simulink model "Demo_TollSystem_cs"  (Simulink 7.6)
settings: Solver=FixedStepDiscrete  SolverMode=SingleTasking  StartTime=0.0  StopTime=13  FixedStep=1/20  RelTol=1e-3
model workspace (MAT data in the model file):
  mbox_table : struct (value not decoded)
  model_closed = 0
  sim_status = 0
PreLoadFcn:
  | check_NUTS_defined
  | model_closed = 0;
  | assignin('base',['model_closed_' bdroot],false);
InitFcn:
  | PreScanExperimentInitFcn(bdroot)
StopFcn:
  | PreScanExperimentStopFcn(bdroot)
libraries: simulink x9, PreScanUsefulBlocks x6, PreScanSimulinkLibrary x4
(part 1 of 2)
CloseFcn:
  | evalin('base',['clear model_closed_' bdroot]);
  | model_closed = 1;
settings Model: Creator=PRESCAN  LastModifiedBy=buildbot
settings OptimizationCC: InitFltsAndDblsToZero=on
settings DebuggingCC: SaveWithParameterizedLinksMsg=none  SignalResolutionControl=TryResolveAllWithWarning  MultiTaskDSMMsg=warning  MultiTaskCondExecSysMsg=none
settings RTWCC: IncludeERTFirstTime=on
settings GRTTargetCC: TargetFcnLib=ansi_tfl_tmw.mat

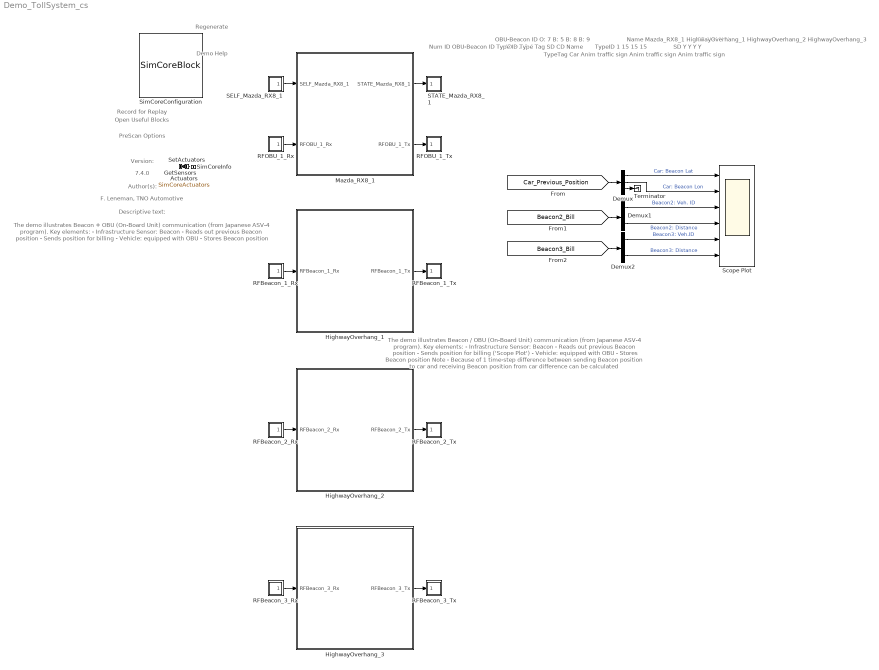
== system Demo_TollSystem_cs ==
  note: The demo illustrates Beacon / OBU (On-Board Unit)
      | communication (from Japanese ASV-4 program).
      |
      | Key elements:
      | - Infrastructure Sensor: Beacon
      |     - Reads out previous Beacon position
      |     - Sends position for billing ('Scope Plot')
      | - Vehicle: equipped with OBU
      |     - Stores Beacon position
      |
      | Note
      | - Because of 1 time-step difference between sending Beacon position
      |   to car and receiving Beacon position from car difference can be
      |   calculated
  note: Demo Help
  note: Regenerate
  note: Record for Replay
  note: Open Useful Blocks
  note: PreScan Options
  note: Version:
  note: 7.4.0
  note: Author(s):
  note: F. Leneman, TNO Automotive
  note: Descriptive text:
  note: The demo illustrates Beacon + OBU
      |
      | (On-Board Unit) communication
      | (from Japanese ASV-4 program).
      |
      | Key elements:
      | - Infrastructure Sensor: Beacon
      |     - Reads out previous Beacon
      | position
      |     - Sends position for billing
      | - Vehicle: equipped with OBU
      |     - Stores Beacon position
  note: ID
      |
      | 6
      | 2
      | 3
      | 4
  note: OBU-Beacon ID
      |
      | O: 7
      | B: 5
      | B: 8
      | B: 9
  note: TypeID
      |
      | 1
      | 15
      | 15
      | 15
  note: TypeTag
      |
      | Car
      | Anim traffic sign
      | Anim traffic sign
      | Anim traffic sign
  note: SD
      |
      | Y
      | Y
      | Y
      | Y
  note: CD
      |
      | N
      | N
      | N
      | N
  note: Name
      |
      | Mazda_RX8_1
      | HighwayOverhang_1
      | HighwayOverhang_2
      | HighwayOverhang_3
  note: Num ID OBU-Beacon ID Type ID Type Tag SD CD Name
  Actuators : DataStoreMemory  Tag=Actuators  DataStoreName=SimCoreActuators  InitialValue=zeros(79,1)
      settings: DeleteFcn=PreScanBlockDeleteFcn;
  Demux : Demux  Outputs=3
  Demux1 : Demux  Outputs=2
  Demux2 : Demux  Outputs=2
  GetSensors : Subsystem  Tag=GetSensors  Priority=2  mask(PreScan Simulation Core Block){NrOfSensors=333, TimeStep=1/20}
      mask prompts: NrOfSensors "Number of sensor values"; TimeStep "Timestep [s]"
      mask help:
      | Please do not remove this block from the PreScan compilation sheet,
      | as it contains essential configuration parameters for a PreScan simulation.
      settings: DeleteFcn=PreScanBlockDeleteFcn;
  HighwayOverhang_1 : Subsystem  Tag=WorldObjectSubSystem  InitFcn=UniqueId = '39';
      mask Display: image(imread('HighwayOverhang.jpg'));color('white');text(0,0,' ID=2\n')
  HighwayOverhang_2 : Subsystem  Tag=WorldObjectSubSystem  InitFcn=UniqueId = '40';
      mask Display: image(imread('HighwayOverhang.jpg'));color('white');text(0,0,' ID=3\n')
  HighwayOverhang_3 : Subsystem  Tag=WorldObjectSubSystem  InitFcn=|
      | UniqueId = '44';
      | UniqueId = '41';
      mask Display: image(imread('HighwayOverhang.jpg'));color('white');text(0,0,' ID=4\n')
  Mazda_RX8_1 : Subsystem  Tag=WorldObjectSubSystem  InitFcn=UniqueId = '16';
      mask Display: image(imread('Mazda_RX8.jpg'));color('white');text(0,0,' ID=6\n')
  RFBeacon_1_Rx : Subsystem  Tag=BeaconRx  Priority=3  mask(PreScan Source Block: Antenna Receiver){NrEntitiesOut=5, PortName=RFBeacon_1, PortIndex=48, PortWidth=95, TimeStep=1/20}
      mask prompts: NrEntitiesOut "User Specified: # of Visible OBUs"; PortName "Auto Assigned: Port Name [-]"; PortIndex "Auto Assigned: Index [-]"; PortWidth "Auto Assigned: Port Dimensions [-]"; TimeStep "Auto Assigned: Upload Period [s]"
      mask help:
      | Using the Beacon and OBU (On-Board Unit) information between actors and infrastructure can be exchanged.
      |
      | The Beacon Reciever receives actor information and user-definable signals.
      |
      | For more information, please click Help.
      settings: DeleteFcn=PreScanBlockDeleteFcn;
      mask Help: eval('openHelp(486)')
      mask Display: image(imread('ico_Beacon_RF_24_gray.png'))
  RFBeacon_1_Tx : Subsystem  Tag=BeaconTx  Priority=0  mask(PreScan Sink Block: AntennaT){PortName=RFBeacon_1, PortIndex=31, PortWidth=16, TimeStep=1/20}
      mask prompts: PortName "Auto Assigned: Port Name [-]"; PortIndex "Auto Assigned: Index [-]"; PortWidth "Auto Assigned: Port Dimensions [-]"; TimeStep "Auto Assigned: Upload Period [s]"
      mask help:
      | Using the Beacon and OBU (On-Board Unit) information between actors and infrastructure can be exchanged.
      |
      | The Beacon Transmitter contains the following, user-definable signals:
      |
      | - Beacon Type		[-]
      | - Spares (1:15)		[-]
      |
      | For more information, please click Help.
      settings: DeleteFcn=PreScanBlockDeleteFcn;
      mask Help: eval('openHelp(486)')
      mask Display: image(imread('ico_Beacon_RF_24_gray.png'))
  RFBeacon_2_Rx : Subsystem  Tag=BeaconRx  Priority=3  mask(PreScan Source Block: Antenna Receiver){NrEntitiesOut=5, PortName=RFBeacon_2, PortIndex=143, PortWidth=95, TimeStep=1/20}
      mask prompts: NrEntitiesOut "User Specified: # of Visible OBUs"; PortName "Auto Assigned: Port Name [-]"; PortIndex "Auto Assigned: Index [-]"; PortWidth "Auto Assigned: Port Dimensions [-]"; TimeStep "Auto Assigned: Upload Period [s]"
      mask help:
      | Using the Beacon and OBU (On-Board Unit) information between actors and infrastructure can be exchanged.
      |
      | The Beacon Reciever receives actor information and user-definable signals.
      |
      | For more information, please click Help.
      settings: DeleteFcn=PreScanBlockDeleteFcn;
      mask Help: eval('openHelp(486)')
      mask Display: image(imread('ico_Beacon_RF_24_gray.png'))
  RFBeacon_2_Tx : Subsystem  Tag=BeaconTx  Priority=0  mask(PreScan Sink Block: AntennaT){PortName=RFBeacon_2, PortIndex=47, PortWidth=16, TimeStep=1/20}
      mask prompts: PortName "Auto Assigned: Port Name [-]"; PortIndex "Auto Assigned: Index [-]"; PortWidth "Auto Assigned: Port Dimensions [-]"; TimeStep "Auto Assigned: Upload Period [s]"
      mask help:
      | Using the Beacon and OBU (On-Board Unit) information between actors and infrastructure can be exchanged.
      |
      | The Beacon Transmitter contains the following, user-definable signals:
      |
      | - Beacon Type		[-]
      | - Spares (1:15)		[-]
      |
      | For more information, please click Help.
      settings: DeleteFcn=PreScanBlockDeleteFcn;
      mask Help: eval('openHelp(486)')
      mask Display: image(imread('ico_Beacon_RF_24_gray.png'))
  RFBeacon_3_Rx : Subsystem  Tag=BeaconRx  Priority=3  mask(PreScan Source Block: Antenna Receiver){NrEntitiesOut=5, PortName=RFBeacon_3, PortIndex=238, PortWidth=95, TimeStep=1/20}
      mask prompts: NrEntitiesOut "User Specified: # of Visible OBUs"; PortName "Auto Assigned: Port Name [-]"; PortIndex "Auto Assigned: Index [-]"; PortWidth "Auto Assigned: Port Dimensions [-]"; TimeStep "Auto Assigned: Upload Period [s]"
      mask help:
      | Using the Beacon and OBU (On-Board Unit) information between actors and infrastructure can be exchanged.
      |
      | The Beacon Reciever receives actor information and user-definable signals.
      |
      | For more information, please click Help.
      settings: DeleteFcn=PreScanBlockDeleteFcn;
      mask Help: eval('openHelp(486)')
      mask Display: image(imread('ico_Beacon_RF_24_gray.png'))
  RFBeacon_3_Tx : Subsystem  Tag=BeaconTx  Priority=0  mask(PreScan Sink Block: AntennaT){PortName=RFBeacon_3, PortIndex=63, PortWidth=16, TimeStep=1/20}
      mask prompts: PortName "Auto Assigned: Port Name [-]"; PortIndex "Auto Assigned: Index [-]"; PortWidth "Auto Assigned: Port Dimensions [-]"; TimeStep "Auto Assigned: Upload Period [s]"
      mask help:
      | Using the Beacon and OBU (On-Board Unit) information between actors and infrastructure can be exchanged.
      |
      | The Beacon Transmitter contains the following, user-definable signals:
      |
      | - Beacon Type		[-]
      | - Spares (1:15)		[-]
      |
      | For more information, please click Help.
      settings: DeleteFcn=PreScanBlockDeleteFcn;
      mask Help: eval('openHelp(486)')
      mask Display: image(imread('ico_Beacon_RF_24_gray.png'))
  RFOBU_1_Rx : Subsystem  Tag=OBURx  Priority=3  mask(PreScan Source Block: Antenna Receiver){NrEntitiesOut=2, PortName=RFOBU_1, PortIndex=8, PortWidth=40, TimeStep=1/20}
      mask prompts: NrEntitiesOut "User Specified: # of Visible OBUs"; PortName "Auto Assigned: Port Name [-]"; PortIndex "Auto Assigned: Index [-]"; PortWidth "Auto Assigned: Port Dimensions [-]"; TimeStep "Auto Assigned: Upload Period [s]"
      mask help:
      | Using the Beacon and OBU (On-Board Unit) information between actors and infrastructure can be exchanged.
      |
      | The OBU Reciever receives infrastructure information and user-definable signals.
      |
      | For more information, please click Help.
      settings: DeleteFcn=PreScanBlockDeleteFcn;
      mask Help: eval('openHelp(487)')
      mask Display: image(imread('ico_OBU_RF_24_gray.png'))
  RFOBU_1_Tx : Subsystem  Tag=OBUTx  Priority=0  mask(PreScan Sink Block: AntennaT){PortName=RFOBU_1, PortIndex=15, PortWidth=16, TimeStep=1/20}
      mask prompts: PortName "Auto Assigned: Port Name [-]"; PortIndex "Auto Assigned: Index [-]"; PortWidth "Auto Assigned: Port Dimensions [-]"; TimeStep "Auto Assigned: Upload Period [s]"
      mask help:
      | Using the Beacon and OBU (On-Board Unit) information between actors and infrastructure can be exchanged.
      |
      | The OBU Transmitter contains the following, user-definable signals:
      |
      | - Vehicle Type		[-]
      | - Spares (1:15)		[-]
      |
      | For more information, please click Help.
      settings: DeleteFcn=PreScanBlockDeleteFcn;
      mask Help: eval('openHelp(487)')
      mask Display: image(imread('ico_OBU_RF_24_gray.png'))
  SELF_Mazda_RX8_1 : Subsystem  Tag=SELF  Priority=3  mask(PreScan Source Block: SELF){PortName=SELF_Mazda_RX8_1, PortIndex=0, PortWidth=8, TimeStep=1/20}
      mask prompts: PortName "Auto-Assigned: Port Name [-]"; PortIndex "Auto-Assigned: Port Index [-]"; PortWidth "Auto-Assigned: Port Dimensions"; TimeStep "Auto-Assigned: Upload Period [s]"
      mask help:
      | The SELF port shows (state) information of the actor itself. The outputs are position in the experiment's axis system and the GPS coordinates, and the object's absolute velocity and compass heading.
      |
      | For more information, please click Help.
      settings: DeleteFcn=PreScanBlockDeleteFcn;
      mask Help: eval('openHelp(462)')
      mask Display: image(imread('GPS.png'))
  STATE_Mazda_RX8_1 : Subsystem  Tag=State  Priority=0  mask(PreScan Sink Block: State){x0=-2.1430611191891602E-16, y0=-1.75, z0=0.51, Roll0=0, Pitch0=0, Yaw0=0, TimeStep=1/20}
      mask prompts: x0 "Ini x-position VEHICLE wrt GLOBAL axis system [m]"; y0 "Ini y-position VEHICLE wrt GLOBAL axis system [m]"; z0 "Ini z-position VEHICLE wrt GLOBAL axis system [m]"; Roll0 "Ini roll-angle BODY wrt VEHICLE axis system [deg]"; Pitch0 "Ini pitch-angle BODY wrt VEHICLE axis system [deg]"; Yaw0 "Ini yaw-angle VEHICLE wrt GLOBAL axis system [deg]"; TimeStep "Time Step [s]"
      mask help:
      | The Actor State contains a vector signal of size (9x1), containing the following signals:
      |
      | -  Position                  (x,y,z)                                     [m]
      | -  Velocity                  (vx,vy,vz)                               [m/s]
      | -  Angles                    (Roll, Pitch, Yaw)                   [rad]
      |
      | The Actor state is defined in the global axis system.
      | The state is superponed on the Initial position defined in the GUI.
      |
      | For more information, please click Help.
      settings: DeleteFcn=PreScanBlockDeleteFcn;
      mask Help: eval('openHelp(222)')
      mask Display: image(imread('State.png'))
  Scope Plot : Scope  NumInputPorts=6
      settings: TimeRange=14  YMin=50~5~0~0~0~0  YMax=55~5.005~200000000000000~100~200000000000000~100
  SetActuators : Subsystem  Tag=SetActuators  Priority=1  mask(PreScan Simulation Core Block){TimeStep=1/20, NrOfActuators=79}
      mask prompts: TimeStep "Timestep [s]"; NrOfActuators "Number of actuator values"
      mask help:
      | Please do not remove this block from the PreScan compilation sheet,
      | as it contains essential configuration parameters for a PreScan simulation.
      settings: DeleteFcn=PreScanBlockDeleteFcn;
  SimCoreConfiguration : M-S-Function  Tag=SimCoreConfiguration  Description=B82875A94833F997F21DD6E9124957973A9674FE07CE9C3E2714F76BA6993981  FunctionName=SimCoreBlock  Parameters=ExperimentXML PortsXML SimulationCore HostName CheckStart EnableLog RfR EnableGPUAccel ShowComputationTime  mask(PreScan Simulation Core Configurator){SimulationCore=NUTS, HostName=0, CheckStart=0, prescanversion='7.4.0', EnableLog=off, RfR=0, EnableGPUAccel=off, ShowComputationTime=off}
      mask prompts: SimulationCore "Simulation Core"; HostName "Simulation Host"; CheckStart "Show START Dialog"; prescanversion "PreScan Version"; EnableLog "Create TA Log"; RfR "Record for Replay"; EnableGPUAccel "Enable GPU Acceleration"; ShowComputationTime "Show ComputationTime Scope"
      mask help:
      | Please do not remove this block from the PreScan compilation sheet,
      | as it contains essential configuration parameter for a PreScan simulation.
      mask init:
      | model = bdroot;
      | ExperimentXML = [model(1:end-3) '.pex'];
      | PortsXML = [model '_ports.pcd'];
      settings: DeleteFcn=PreScanBlockDeleteFcn;  ModelCloseFcn=assignin('base',['model_closed_' bdroot],true);
      mask Help: eval('openHelp(812)')
      mask Display: image(imread('prescanlogo.ico'))
  SimCoreInfo : Subsystem  Tag=SimCoreInfo
  Terminator : Terminator
  wires:
  [Car_Previous_Position] -> Demux/1
  Demux/3 -> Terminator/1
  Demux/1 -> Scope Plot/1  "Car: Beacon Lat"
  Demux/2 -> Scope Plot/2  "Car: Beacon Lon"
  [Beacon2_Bill] -> Demux1/1
  Demux1/1 -> Scope Plot/3  "Beacon2: Veh. ID"
  Demux1/2 -> Scope Plot/4  "Beacon2: Distance"
  [Beacon3_Bill] -> Demux2/1
  Demux2/1 -> Scope Plot/5  "Beacon3: Veh.ID"
  Demux2/2 -> Scope Plot/6  "Beacon3: Distance"
  Mazda_RX8_1/1(STATE_Mazda_RX8_1) -> STATE_Mazda_RX8_1/1(State)
  SELF_Mazda_RX8_1/1(U) -> Mazda_RX8_1/1(SELF_Mazda_RX8_1)
  RFOBU_1_Rx/1(U) -> Mazda_RX8_1/2(RFOBU_1_Rx)
  Mazda_RX8_1/2(RFOBU_1_Tx) -> RFOBU_1_Tx/1(Y)
  RFBeacon_1_Rx/1(U) -> HighwayOverhang_1/1(RFBeacon_1_Rx)
  HighwayOverhang_1/1(RFBeacon_1_Tx) -> RFBeacon_1_Tx/1(Y)
  RFBeacon_2_Rx/1(U) -> HighwayOverhang_2/1(RFBeacon_2_Rx)
  HighwayOverhang_2/1(RFBeacon_2_Tx) -> RFBeacon_2_Tx/1(Y)
  RFBeacon_3_Rx/1(U) -> HighwayOverhang_3/1(RFBeacon_3_Rx)
  HighwayOverhang_3/1(RFBeacon_3_Tx) -> RFBeacon_3_Tx/1(Y)
  SetActuators/1(dummy) -> GetSensors/1(dummy)

== system Demo_TollSystem_cs/GetSensors ==
  dummy : Inport
  GetSensors : M-S-Function  FunctionName=GetSensorsBlock  Parameters=TimeStep NrOfSensors
  tag scope: SimCoreSensors=global
  wires:
  GetSensors/1 -> [SimCoreSensors]
  dummy/1 -> GetSensors/1

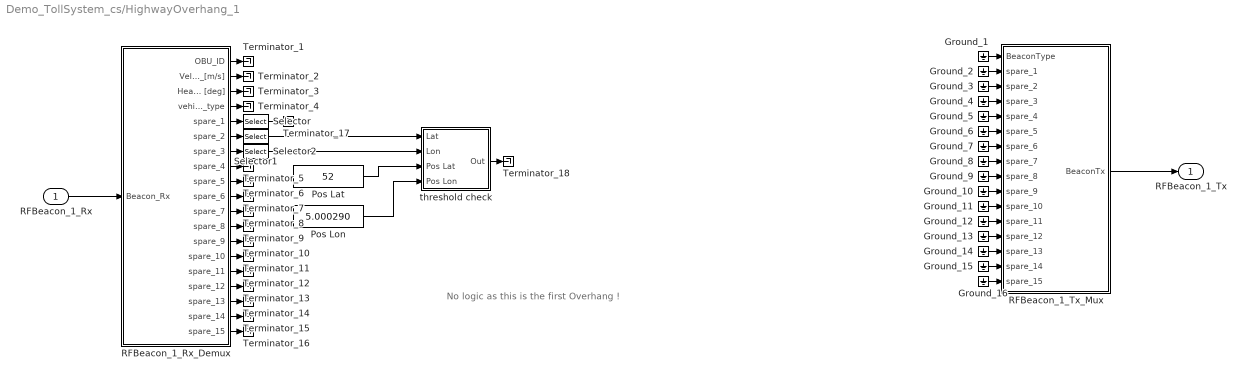
== system Demo_TollSystem_cs/HighwayOverhang_1 ==
  note: No logic as this is the first Overhang !
  RFBeacon_1_Rx : Inport  Tag=BeaconRxInport
  Ground_{1..16} (16 alike) : Ground
  Pos Lat : Constant  Value=52
  Pos Lon : Constant  Value=5.000290
  RFBeacon_1_Rx_Demux : Subsystem  Tag=DemuxAntennaR  mask(PreScan Demux Block:){Technology='RF'}
      mask init:
      | IconTxt = char('','','','','Technology:            ',['{\it',Technology,'}']);
      settings: DeleteFcn=PreScanBlockDeleteFcn;
      mask Display:
      | disp(IconTxt,'texmode','on')
      | port_label('output', 1, 'OBU ID [-]')
      | port_label('output', 2, 'OBU Velocity [m/s]')
      | port_label('output', 3, 'OBU Heading [deg]')
      | port_label('output', 4, 'Vehicle Type[-]')
      | port_label('output', 5, 'Veh. Reg.')
      | port_label('output', 6, 'Previous pos. - Lat')
      | port_label('output', 7, 'Previous pos. - Lon')
      | port_label('output', 8, 'Previous pos. - Alt')
      | port_label('output', 9, 'spare_5')
      | port_label('output', 10, 'spare_6')
      | port_label('output', 11, 'spare_7')
      | port_label('output', 12, 'spare_8')
      | port_label('output', 13, 'spare_9')
      | port_label('output', 14, 'spare_10')
      | port_label('output', 15, 'spare_11')
      | port_label('output', 16, 'spare_12')
      | port_label('output', 17, 'spare_13')
      | port_label('output', 18, 'spare_14')
      | port_label('output', 19, 'spare_15')
  RFBeacon_1_Tx_Mux : Subsystem  Tag=MuxBeaconTx  mask(PreScan Mux Block:){Technology='RF'}
      mask init:
      | IconTxt = char('','','','              Technology:',['{\it                ',Technology,'}']);
      settings: DeleteFcn=PreScanBlockDeleteFcn;
      mask Display:
      | disp(IconTxt,'texmode','on')
      | port_label('input', 1, 'Beacon Type [-]')
      | port_label('input', 2, 'spare_1')
      | port_label('input', 3, 'spare_2')
      | port_label('input', 4, 'spare_3')
      | port_label('input', 5, 'spare_4')
      | port_label('input', 6, 'spare_5')
      | port_label('input', 7, 'spare_6')
      | port_label('input', 8, 'spare_7')
      | port_label('input', 9, 'spare_8')
      | port_label('input', 10, 'spare_9')
      | port_label('input', 11, 'spare_10')
      | port_label('input', 12, 'spare_11')
      | port_label('input', 13, 'spare_12')
      | port_label('input', 14, 'spare_13')
      | port_label('input', 15, 'spare_14')
      | port_label('input', 16, 'spare_15')
  Selector : Selector  IndexOptions=Index vector (dialog)  Indices=[1]  OutputSizes=1
  Selector1 : Selector  IndexOptions=Index vector (dialog)  Indices=[1]  OutputSizes=1
  Selector2 : Selector  IndexOptions=Index vector (dialog)  Indices=[1]  OutputSizes=1
  Terminator_{1..18} (18 alike) : Terminator
  threshold check : Subsystem
  RFBeacon_1_Tx : Outport  Tag=AntennaTOutport
  wires:
  Selector1/1 -> threshold check/1(Lat)
  Selector2/1 -> threshold check/2(Lon)
  Pos Lat/1 -> threshold check/3(Pos Lat)
  Pos Lon/1 -> threshold check/4(Pos Lon)
  RFBeacon_1_Rx/1 -> RFBeacon_1_Rx_Demux/1(Beacon_Rx)
  RFBeacon_1_Tx_Mux/1(BeaconTx) -> RFBeacon_1_Tx/1
  RFBeacon_1_Rx_Demux/5(spare_1) -> Selector/1
  RFBeacon_1_Rx_Demux/6(spare_2) -> Selector1/1
  RFBeacon_1_Rx_Demux/7(spare_3) -> Selector2/1
  RFBeacon_1_Rx_Demux/1(OBU_ID) -> Terminator_1/1
  RFBeacon_1_Rx_Demux/2(Velocity_[m/s]) -> Terminator_2/1
  RFBeacon_1_Rx_Demux/3(Heading [deg]) -> Terminator_3/1
  RFBeacon_1_Rx_Demux/4(vehicle_type) -> Terminator_4/1
  RFBeacon_1_Rx_Demux/8(spare_4) -> Terminator_5/1
  RFBeacon_1_Rx_Demux/9(spare_5) -> Terminator_6/1
  RFBeacon_1_Rx_Demux/10(spare_6) -> Terminator_7/1
  RFBeacon_1_Rx_Demux/11(spare_7) -> Terminator_8/1
  RFBeacon_1_Rx_Demux/12(spare_8) -> Terminator_9/1
  RFBeacon_1_Rx_Demux/13(spare_9) -> Terminator_10/1
  RFBeacon_1_Rx_Demux/14(spare_10) -> Terminator_11/1
  RFBeacon_1_Rx_Demux/15(spare_11) -> Terminator_12/1
  RFBeacon_1_Rx_Demux/16(spare_12) -> Terminator_13/1
  RFBeacon_1_Rx_Demux/17(spare_13) -> Terminator_14/1
  RFBeacon_1_Rx_Demux/18(spare_14) -> Terminator_15/1
  RFBeacon_1_Rx_Demux/19(spare_15) -> Terminator_16/1
  Ground_1/1 -> RFBeacon_1_Tx_Mux/1(BeaconType)
  Ground_2/1 -> RFBeacon_1_Tx_Mux/2(spare_1)
  Ground_3/1 -> RFBeacon_1_Tx_Mux/3(spare_2)
  Ground_4/1 -> RFBeacon_1_Tx_Mux/4(spare_3)
  Ground_5/1 -> RFBeacon_1_Tx_Mux/5(spare_4)
  Ground_6/1 -> RFBeacon_1_Tx_Mux/6(spare_5)
  Ground_7/1 -> RFBeacon_1_Tx_Mux/7(spare_6)
  Ground_8/1 -> RFBeacon_1_Tx_Mux/8(spare_7)
  Ground_9/1 -> RFBeacon_1_Tx_Mux/9(spare_8)
  Ground_10/1 -> RFBeacon_1_Tx_Mux/10(spare_9)
  Ground_11/1 -> RFBeacon_1_Tx_Mux/11(spare_10)
  Ground_12/1 -> RFBeacon_1_Tx_Mux/12(spare_11)
  Ground_13/1 -> RFBeacon_1_Tx_Mux/13(spare_12)
  Ground_14/1 -> RFBeacon_1_Tx_Mux/14(spare_13)
  Ground_15/1 -> RFBeacon_1_Tx_Mux/15(spare_14)
  Ground_16/1 -> RFBeacon_1_Tx_Mux/16(spare_15)
  Selector/1 -> Terminator_17/1
  threshold check/1(Out) -> Terminator_18/1

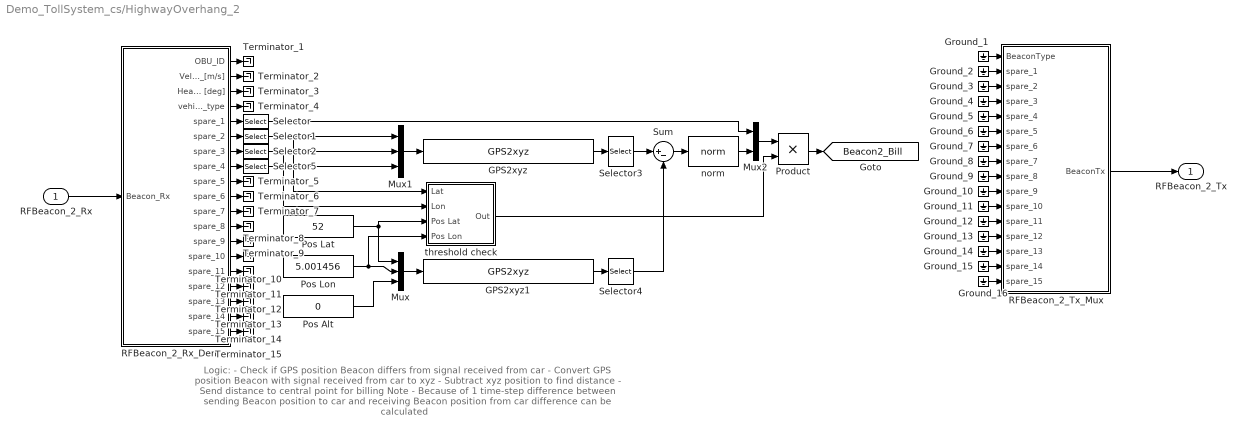
== system Demo_TollSystem_cs/HighwayOverhang_2 ==
  note: Logic:
      | - Check if GPS position Beacon differs from signal received from car
      | - Convert GPS position Beacon with signal received from car to xyz
      | - Subtract xyz position to find distance
      | - Send distance to central point for billing
      |
      | Note
      | - Because of 1 time-step difference between sending Beacon position
      |   to car and receiving Beacon position from car difference can be
      |   calculated
  RFBeacon_2_Rx : Inport  Tag=BeaconRxInport
  GPS2xyz : PreScanUsefulBlocks/GPS2xyz  CoordinateCount=1  GPS_base=[52 5 0]
  GPS2xyz1 : PreScanUsefulBlocks/GPS2xyz  CoordinateCount=1  GPS_base=[52 5 0]
  Ground_{1..16} (16 alike) : Ground
  Mux : Mux  Inputs=3
  Mux1 : Mux  Inputs=3
  Mux2 : Mux  Inputs=2
  Pos Alt : Constant  Value=0
  Pos Lat : Constant  Value=52
  Pos Lon : Constant  Value=5.001456
  Product : Product  RndMeth=Zero
  RFBeacon_2_Rx_Demux : Subsystem  Tag=DemuxAntennaR  mask(PreScan Demux Block:){Technology='RF'}
      mask init:
      | IconTxt = char('','','','','Technology:            ',['{\it',Technology,'}']);
      settings: DeleteFcn=PreScanBlockDeleteFcn;
      mask Display:
      | disp(IconTxt,'texmode','on')
      | port_label('output', 1, 'OBU ID [-]')
      | port_label('output', 2, 'OBU Velocity [m/s]')
      | port_label('output', 3, 'OBU Heading [deg]')
      | port_label('output', 4, 'Vehicle Type[-]')
      | port_label('output', 5, 'Veh. Reg.')
      | port_label('output', 6, 'Previous pos. - Lat')
      | port_label('output', 7, 'Previous pos. - Lon')
      | port_label('output', 8, 'Previous pos. - Alt')
      | port_label('output', 9, 'spare_5')
      | port_label('output', 10, 'spare_6')
      | port_label('output', 11, 'spare_7')
      | port_label('output', 12, 'spare_8')
      | port_label('output', 13, 'spare_9')
      | port_label('output', 14, 'spare_10')
      | port_label('output', 15, 'spare_11')
      | port_label('output', 16, 'spare_12')
      | port_label('output', 17, 'spare_13')
      | port_label('output', 18, 'spare_14')
      | port_label('output', 19, 'spare_15')
  RFBeacon_2_Tx_Mux : Subsystem  Tag=MuxBeaconTx  mask(PreScan Mux Block:){Technology='RF'}
      mask init:
      | IconTxt = char('','','','              Technology:',['{\it                ',Technology,'}']);
      settings: DeleteFcn=PreScanBlockDeleteFcn;
      mask Display:
      | disp(IconTxt,'texmode','on')
      | port_label('input', 1, 'Beacon Type [-]')
      | port_label('input', 2, 'spare_1')
      | port_label('input', 3, 'spare_2')
      | port_label('input', 4, 'spare_3')
      | port_label('input', 5, 'spare_4')
      | port_label('input', 6, 'spare_5')
      | port_label('input', 7, 'spare_6')
      | port_label('input', 8, 'spare_7')
      | port_label('input', 9, 'spare_8')
      | port_label('input', 10, 'spare_9')
      | port_label('input', 11, 'spare_10')
      | port_label('input', 12, 'spare_11')
      | port_label('input', 13, 'spare_12')
      | port_label('input', 14, 'spare_13')
      | port_label('input', 15, 'spare_14')
      | port_label('input', 16, 'spare_15')
  Selector{,1..2,5} (4 alike) : Selector  IndexOptions=Index vector (dialog)  Indices=[1]  OutputSizes=1
  Selector3 : Selector  InputPortWidth=3  IndexOptions=Index vector (dialog)  Indices=[1 2]  OutputSizes=1
  Selector4 : Selector  InputPortWidth=3  IndexOptions=Index vector (dialog)  Indices=[1 2]  OutputSizes=1
  Sum : Sum  Inputs=|+-
  Terminator_{1..15} (15 alike) : Terminator
  norm : MATLABFcn  MATLABFcn=norm
  threshold check : Subsystem
  RFBeacon_2_Tx : Outport  Tag=AntennaTOutport
  tag scope: Beacon2_Bill=global
  wires:
  threshold check/1(Out) -> Product/2
  Pos Lat/1 -> threshold check/3(Pos Lat), Mux/1
  Pos Lon/1 -> threshold check/4(Pos Lon), Mux/2
  Pos Alt/1 -> Mux/3
  Selector/1 -> Mux2/1
  Selector1/1 -> threshold check/1(Lat), Mux1/1
  Selector2/1 -> Mux1/2, threshold check/2(Lon)
  Mux1/1 -> GPS2xyz/1
  Mux/1 -> GPS2xyz1/1
  GPS2xyz/1 -> Selector3/1
  GPS2xyz1/1 -> Selector4/1
  Selector3/1 -> Sum/1
  Selector4/1 -> Sum/2
  Sum/1 -> norm/1
  Selector5/1 -> Mux1/3
  norm/1 -> Mux2/2
  Mux2/1 -> Product/1
  Product/1 -> [Beacon2_Bill]
  RFBeacon_2_Rx/1 -> RFBeacon_2_Rx_Demux/1(Beacon_Rx)
  RFBeacon_2_Tx_Mux/1(BeaconTx) -> RFBeacon_2_Tx/1
  RFBeacon_2_Rx_Demux/5(spare_1) -> Selector/1
  RFBeacon_2_Rx_Demux/6(spare_2) -> Selector1/1
  RFBeacon_2_Rx_Demux/7(spare_3) -> Selector2/1
  RFBeacon_2_Rx_Demux/8(spare_4) -> Selector5/1
  RFBeacon_2_Rx_Demux/1(OBU_ID) -> Terminator_1/1
  RFBeacon_2_Rx_Demux/2(Velocity_[m/s]) -> Terminator_2/1
  RFBeacon_2_Rx_Demux/3(Heading [deg]) -> Terminator_3/1
  RFBeacon_2_Rx_Demux/4(vehicle_type) -> Terminator_4/1
  RFBeacon_2_Rx_Demux/9(spare_5) -> Terminator_5/1
  RFBeacon_2_Rx_Demux/10(spare_6) -> Terminator_6/1
  RFBeacon_2_Rx_Demux/11(spare_7) -> Terminator_7/1
  RFBeacon_2_Rx_Demux/12(spare_8) -> Terminator_8/1
  RFBeacon_2_Rx_Demux/13(spare_9) -> Terminator_9/1
  RFBeacon_2_Rx_Demux/14(spare_10) -> Terminator_10/1
  RFBeacon_2_Rx_Demux/15(spare_11) -> Terminator_11/1
  RFBeacon_2_Rx_Demux/16(spare_12) -> Terminator_12/1
  RFBeacon_2_Rx_Demux/17(spare_13) -> Terminator_13/1
  RFBeacon_2_Rx_Demux/18(spare_14) -> Terminator_14/1
  RFBeacon_2_Rx_Demux/19(spare_15) -> Terminator_15/1
  Ground_1/1 -> RFBeacon_2_Tx_Mux/1(BeaconType)
  Ground_2/1 -> RFBeacon_2_Tx_Mux/2(spare_1)
  Ground_3/1 -> RFBeacon_2_Tx_Mux/3(spare_2)
  Ground_4/1 -> RFBeacon_2_Tx_Mux/4(spare_3)
  Ground_5/1 -> RFBeacon_2_Tx_Mux/5(spare_4)
  Ground_6/1 -> RFBeacon_2_Tx_Mux/6(spare_5)
  Ground_7/1 -> RFBeacon_2_Tx_Mux/7(spare_6)
  Ground_8/1 -> RFBeacon_2_Tx_Mux/8(spare_7)
  Ground_9/1 -> RFBeacon_2_Tx_Mux/9(spare_8)
  Ground_10/1 -> RFBeacon_2_Tx_Mux/10(spare_9)
  Ground_11/1 -> RFBeacon_2_Tx_Mux/11(spare_10)
  Ground_12/1 -> RFBeacon_2_Tx_Mux/12(spare_11)
  Ground_13/1 -> RFBeacon_2_Tx_Mux/13(spare_12)
  Ground_14/1 -> RFBeacon_2_Tx_Mux/14(spare_13)
  Ground_15/1 -> RFBeacon_2_Tx_Mux/15(spare_14)
  Ground_16/1 -> RFBeacon_2_Tx_Mux/16(spare_15)

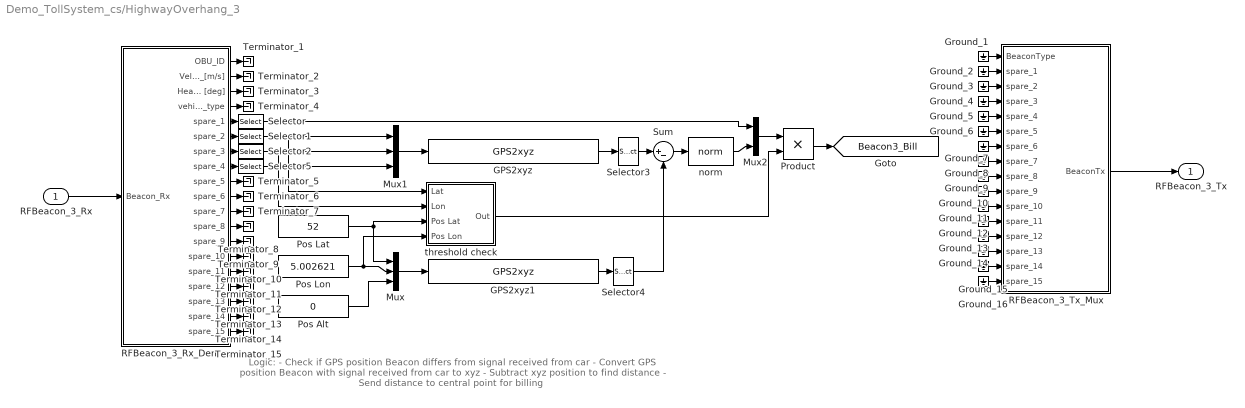
== system Demo_TollSystem_cs/HighwayOverhang_3 ==
  note: Logic:
      | - Check if GPS position Beacon differs from signal received from car
      | - Convert GPS position Beacon with signal received from car to xyz
      | - Subtract xyz position to find distance
      | - Send distance to central point for billing
  RFBeacon_3_Rx : Inport  Tag=BeaconRxInport
  GPS2xyz : PreScanUsefulBlocks/GPS2xyz  CoordinateCount=1  GPS_base=[52 5 0]
  GPS2xyz1 : PreScanUsefulBlocks/GPS2xyz  CoordinateCount=1  GPS_base=[52 5 0]
  Ground_{1..16} (16 alike) : Ground
  Mux : Mux  Inputs=3
  Mux1 : Mux  Inputs=3
  Mux2 : Mux  Inputs=2
  Pos Alt : Constant  Value=0
  Pos Lat : Constant  Value=52
  Pos Lon : Constant  Value=5.002621
  Product : Product  RndMeth=Zero
  RFBeacon_3_Rx_Demux : Subsystem  Tag=DemuxAntennaR  mask(PreScan Demux Block:){Technology='RF'}
      mask init:
      | IconTxt = char('','','','','Technology:            ',['{\it',Technology,'}']);
      settings: DeleteFcn=PreScanBlockDeleteFcn;
      mask Display:
      | disp(IconTxt,'texmode','on')
      | port_label('output', 1, 'OBU ID [-]')
      | port_label('output', 2, 'OBU Velocity [m/s]')
      | port_label('output', 3, 'OBU Heading [deg]')
      | port_label('output', 4, 'Vehicle Type[-]')
      | port_label('output', 5, 'Veh. Reg.')
      | port_label('output', 6, 'Previous pos. - Lat')
      | port_label('output', 7, 'Previous pos. - Lon')
      | port_label('output', 8, 'Previous pos. - Alt')
      | port_label('output', 9, 'spare_5')
      | port_label('output', 10, 'spare_6')
      | port_label('output', 11, 'spare_7')
      | port_label('output', 12, 'spare_8')
      | port_label('output', 13, 'spare_9')
      | port_label('output', 14, 'spare_10')
      | port_label('output', 15, 'spare_11')
      | port_label('output', 16, 'spare_12')
      | port_label('output', 17, 'spare_13')
      | port_label('output', 18, 'spare_14')
      | port_label('output', 19, 'spare_15')
  RFBeacon_3_Tx_Mux : Subsystem  Tag=MuxBeaconTx  mask(PreScan Mux Block:){Technology='RF'}
      mask init:
      | IconTxt = char('','','','              Technology:',['{\it                ',Technology,'}']);
      settings: DeleteFcn=PreScanBlockDeleteFcn;
      mask Display:
      | disp(IconTxt,'texmode','on')
      | port_label('input', 1, 'Beacon Type [-]')
      | port_label('input', 2, 'spare_1')
      | port_label('input', 3, 'spare_2')
      | port_label('input', 4, 'spare_3')
      | port_label('input', 5, 'spare_4')
      | port_label('input', 6, 'spare_5')
      | port_label('input', 7, 'spare_6')
      | port_label('input', 8, 'spare_7')
      | port_label('input', 9, 'spare_8')
      | port_label('input', 10, 'spare_9')
      | port_label('input', 11, 'spare_10')
      | port_label('input', 12, 'spare_11')
      | port_label('input', 13, 'spare_12')
      | port_label('input', 14, 'spare_13')
      | port_label('input', 15, 'spare_14')
      | port_label('input', 16, 'spare_15')
  Selector{,1..2,5} (4 alike) : Selector  IndexOptions=Index vector (dialog)  Indices=[1]  OutputSizes=1
  Selector3 : Selector  InputPortWidth=3  IndexOptions=Index vector (dialog)  Indices=[1 2]  OutputSizes=1
  Selector4 : Selector  InputPortWidth=3  IndexOptions=Index vector (dialog)  Indices=[1 2]  OutputSizes=1
  Sum : Sum  Inputs=|+-
  Terminator_{1..15} (15 alike) : Terminator
  norm : MATLABFcn  MATLABFcn=norm
  threshold check : Subsystem
  RFBeacon_3_Tx : Outport  Tag=AntennaTOutport
  tag scope: Beacon3_Bill=global
  wires:
  threshold check/1(Out) -> Product/2
  Pos Lat/1 -> threshold check/3(Pos Lat), Mux/1
  Pos Lon/1 -> threshold check/4(Pos Lon), Mux/2
  Pos Alt/1 -> Mux/3
  Selector/1 -> Mux2/1
  Selector1/1 -> threshold check/1(Lat), Mux1/1
  Selector2/1 -> Mux1/2, threshold check/2(Lon)
  Mux1/1 -> GPS2xyz/1
  Mux/1 -> GPS2xyz1/1
  GPS2xyz/1 -> Selector3/1
  GPS2xyz1/1 -> Selector4/1
  Selector3/1 -> Sum/1
  Selector4/1 -> Sum/2
  Sum/1 -> norm/1
  Selector5/1 -> Mux1/3
  norm/1 -> Mux2/2
  Mux2/1 -> Product/1
  Product/1 -> [Beacon3_Bill]
  RFBeacon_3_Rx/1 -> RFBeacon_3_Rx_Demux/1(Beacon_Rx)
  RFBeacon_3_Tx_Mux/1(BeaconTx) -> RFBeacon_3_Tx/1
  RFBeacon_3_Rx_Demux/5(spare_1) -> Selector/1
  RFBeacon_3_Rx_Demux/6(spare_2) -> Selector1/1
  RFBeacon_3_Rx_Demux/7(spare_3) -> Selector2/1
  RFBeacon_3_Rx_Demux/8(spare_4) -> Selector5/1
  RFBeacon_3_Rx_Demux/1(OBU_ID) -> Terminator_1/1
  RFBeacon_3_Rx_Demux/2(Velocity_[m/s]) -> Terminator_2/1
  RFBeacon_3_Rx_Demux/3(Heading [deg]) -> Terminator_3/1
  RFBeacon_3_Rx_Demux/4(vehicle_type) -> Terminator_4/1
  RFBeacon_3_Rx_Demux/9(spare_5) -> Terminator_5/1
  RFBeacon_3_Rx_Demux/10(spare_6) -> Terminator_6/1
  RFBeacon_3_Rx_Demux/11(spare_7) -> Terminator_7/1
  RFBeacon_3_Rx_Demux/12(spare_8) -> Terminator_8/1
  RFBeacon_3_Rx_Demux/13(spare_9) -> Terminator_9/1
  RFBeacon_3_Rx_Demux/14(spare_10) -> Terminator_10/1
  RFBeacon_3_Rx_Demux/15(spare_11) -> Terminator_11/1
  RFBeacon_3_Rx_Demux/16(spare_12) -> Terminator_12/1
  RFBeacon_3_Rx_Demux/17(spare_13) -> Terminator_13/1
  RFBeacon_3_Rx_Demux/18(spare_14) -> Terminator_14/1
  RFBeacon_3_Rx_Demux/19(spare_15) -> Terminator_15/1
  Ground_1/1 -> RFBeacon_3_Tx_Mux/1(BeaconType)
  Ground_2/1 -> RFBeacon_3_Tx_Mux/2(spare_1)
  Ground_3/1 -> RFBeacon_3_Tx_Mux/3(spare_2)
  Ground_4/1 -> RFBeacon_3_Tx_Mux/4(spare_3)
  Ground_5/1 -> RFBeacon_3_Tx_Mux/5(spare_4)
  Ground_6/1 -> RFBeacon_3_Tx_Mux/6(spare_5)
  Ground_7/1 -> RFBeacon_3_Tx_Mux/7(spare_6)
  Ground_8/1 -> RFBeacon_3_Tx_Mux/8(spare_7)
  Ground_9/1 -> RFBeacon_3_Tx_Mux/9(spare_8)
  Ground_10/1 -> RFBeacon_3_Tx_Mux/10(spare_9)
  Ground_11/1 -> RFBeacon_3_Tx_Mux/11(spare_10)
  Ground_12/1 -> RFBeacon_3_Tx_Mux/12(spare_11)
  Ground_13/1 -> RFBeacon_3_Tx_Mux/13(spare_12)
  Ground_14/1 -> RFBeacon_3_Tx_Mux/14(spare_13)
  Ground_15/1 -> RFBeacon_3_Tx_Mux/15(spare_14)
  Ground_16/1 -> RFBeacon_3_Tx_Mux/16(spare_15)

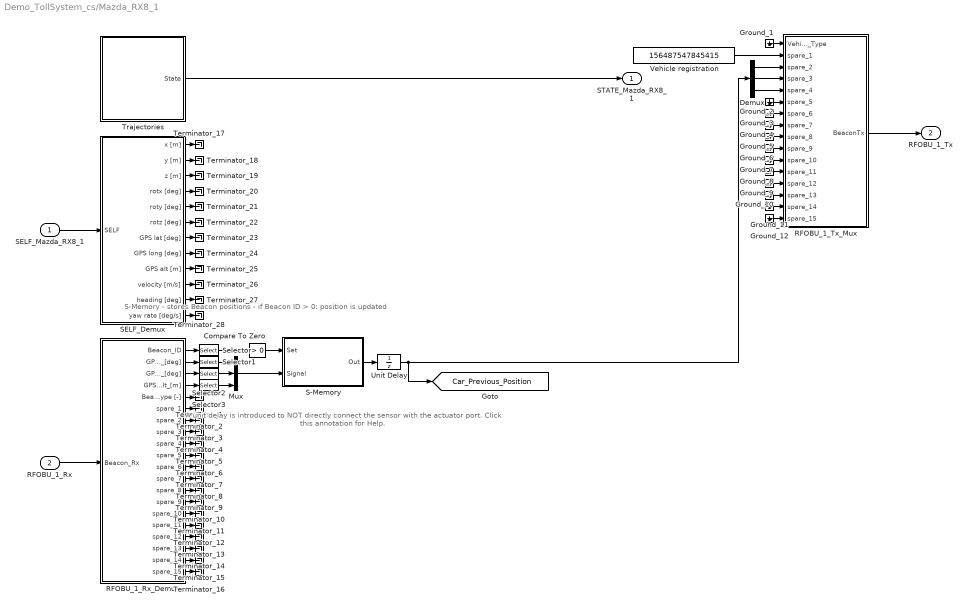
== system Demo_TollSystem_cs/Mazda_RX8_1 ==
  note: A unit delay is introduced to NOT
      | directly connect the sensor with
      | the actuator port.
      |
      | Click this annotation for Help.
  note: S-Memory
      | - stores Beacon positions
      | - if Beacon ID > 0: position is updated
  SELF_Mazda_RX8_1 : Inport  Tag=SELFInport
  RFOBU_1_Rx : Inport  Tag=OBURxInport  Port=2
  Compare To Zero : simulink/Logic and Bit Operations/Compare To Zero  SystemSampleTime=-1  relop=>  LogicOutDataTypeMode=uint8  ZeroCross=off
  Demux : Demux  Outputs=3
  Ground_{1..12} (12 alike) : Ground
  Mux : Mux  Inputs=3
  RFOBU_1_Rx_Demux : Subsystem  Tag=DemuxOBURx  mask(PreScan Demux Block:){Technology='RF'}
      mask init:
      | IconTxt = char('','','','Technology:            ',['{\it',Technology,'}']);
      settings: DeleteFcn=PreScanBlockDeleteFcn;
      mask Display:
      | disp(IconTxt,'texmode','on')
      | port_label('output', 1, 'Beacon ID [-]')
      | port_label('output', 2, 'Beacon GPS Lat [deg]')
      | port_label('output', 3, 'Beacon GPS Lon [deg]')
      | port_label('output', 4, 'Beacon GPS Alt [m]')
      | port_label('output', 5, 'BeaconType [-]')
      | port_label('output', 6, 'spare_1')
      | port_label('output', 7, 'spare_2')
      | port_label('output', 8, 'spare_3')
      | port_label('output', 9, 'spare_4')
      | port_label('output', 10, 'spare_5')
      | port_label('output', 11, 'spare_6')
      | port_label('output', 12, 'spare_7')
      | port_label('output', 13, 'spare_8')
      | port_label('output', 14, 'spare_9')
      | port_label('output', 15, 'spare_10')
      | port_label('output', 16, 'spare_11')
      | port_label('output', 17, 'spare_12')
      | port_label('output', 18, 'spare_13')
      | port_label('output', 19, 'spare_14')
      | port_label('output', 20, 'spare_15')
  RFOBU_1_Tx_Mux : Subsystem  Tag=MuxOBUTx  mask(PreScan Mux Block:){Technology='RF'}
      mask init:
      | IconTxt = char('','','              Technology:',['{\it                ',Technology,'}']);
      settings: DeleteFcn=PreScanBlockDeleteFcn;
      mask Display:
      | disp(IconTxt,'texmode','on')
      | port_label('input', 1, 'Vehicle Type [-]')
      | port_label('input', 2, 'Veh. Reg.')
      | port_label('input', 3, 'Previous pos. - Lat')
      | port_label('input', 4, 'Previous pos. - Lon')
      | port_label('input', 5, 'Previous pos. - Alt')
      | port_label('input', 6, 'spare_5')
      | port_label('input', 7, 'spare_6')
      | port_label('input', 8, 'spare_7')
      | port_label('input', 9, 'spare_8')
      | port_label('input', 10, 'spare_9')
      | port_label('input', 11, 'spare_10')
      | port_label('input', 12, 'spare_11')
      | port_label('input', 13, 'spare_12')
      | port_label('input', 14, 'spare_13')
      | port_label('input', 15, 'spare_14')
      | port_label('input', 16, 'spare_15')
  S-Memory : Subsystem
  SELF_Demux : Subsystem  Tag=DemuxSELF
      settings: DeleteFcn=PreScanBlockDeleteFcn;
      mask Type: PreScan Demux Block:
      mask Display:
      | port_label('output',1,'x [m]')
      | port_label('output',2,'y [m]')
      | port_label('output',3,'z [m]','texmode','on')
      | port_label('output',4,'Rotx [deg]','texmode','on')
      | port_label('output',5,'Roty [deg]','texmode','on')
      | port_label('output',6,'Rotz [deg]','texmode','on')
      | port_label('output',7,'GPS lat [deg]','texmode','on')
      | port_label('output',8,'GPS long [deg]','texmode','on')
      | port_label('output',9,'GPS alt [m]','texmode','on')
      | port_label('output',10,'Velocity [m/s]')
      | port_label('output',11,'Heading [deg]')
      | port_label('output',12,'Yaw rate [deg/s]')
  Selector{,1..3} (4 alike) : Selector  IndexOptions=Index vector (dialog)  Indices=[1]  OutputSizes=1
  Terminator_{1..28} (28 alike) : Terminator
  Trajectories : Subsystem  Tag=Trajectories
      mask Display: image(imread('Trajectory.png'));
  Unit Delay : UnitDelay  SampleTime=-1
  Vehicle registration : Constant  Value=156487547845415
  STATE_Mazda_RX8_1 : Outport  Tag=StateOutport
  RFOBU_1_Tx : Outport  Tag=AntennaTOutport  Port=2
  tag scope: Car_Previous_Position=global
  wires:
  Mux/1 -> S-Memory/2(Signal)
  Compare To Zero/1 -> S-Memory/1(Set)
  Selector/1 -> Compare To Zero/1
  Selector1/1 -> Mux/1
  Selector2/1 -> Mux/2
  S-Memory/1(Out) -> Unit Delay/1
  Selector3/1 -> Mux/3
  Unit Delay/1 -> Demux/1, [Car_Previous_Position]
  SELF_Mazda_RX8_1/1 -> SELF_Demux/1(SELF)
  RFOBU_1_Rx/1 -> RFOBU_1_Rx_Demux/1(Beacon_Rx)
  RFOBU_1_Tx_Mux/1(BeaconTx) -> RFOBU_1_Tx/1
  Trajectories/1(State) -> STATE_Mazda_RX8_1/1
  RFOBU_1_Rx_Demux/1(Beacon_ID) -> Selector/1
  RFOBU_1_Rx_Demux/2(GPS_pos_lat_[deg]) -> Selector1/1
  RFOBU_1_Rx_Demux/3(GPS_pos_long_[deg]) -> Selector2/1
  Vehicle registration/1 -> RFOBU_1_Tx_Mux/2(spare_1)
  Demux/1 -> RFOBU_1_Tx_Mux/3(spare_2)
  Demux/2 -> RFOBU_1_Tx_Mux/4(spare_3)
  RFOBU_1_Rx_Demux/4(GPS_pos_alt_[m]) -> Selector3/1
  Demux/3 -> RFOBU_1_Tx_Mux/5(spare_4)
  RFOBU_1_Rx_Demux/5(BeaconType [-]) -> Terminator_1/1
  RFOBU_1_Rx_Demux/6(spare_1) -> Terminator_2/1
  RFOBU_1_Rx_Demux/7(spare_2) -> Terminator_3/1
  RFOBU_1_Rx_Demux/8(spare_3) -> Terminator_4/1
  RFOBU_1_Rx_Demux/9(spare_4) -> Terminator_5/1
  RFOBU_1_Rx_Demux/10(spare_5) -> Terminator_6/1
  RFOBU_1_Rx_Demux/11(spare_6) -> Terminator_7/1
  RFOBU_1_Rx_Demux/12(spare_7) -> Terminator_8/1
  RFOBU_1_Rx_Demux/13(spare_8) -> Terminator_9/1
  RFOBU_1_Rx_Demux/14(spare_9) -> Terminator_10/1
  RFOBU_1_Rx_Demux/15(spare_10) -> Terminator_11/1
  RFOBU_1_Rx_Demux/16(spare_11) -> Terminator_12/1
  RFOBU_1_Rx_Demux/17(spare_12) -> Terminator_13/1
  RFOBU_1_Rx_Demux/18(spare_13) -> Terminator_14/1
  RFOBU_1_Rx_Demux/19(spare_14) -> Terminator_15/1
  RFOBU_1_Rx_Demux/20(spare_15) -> Terminator_16/1
  Ground_1/1 -> RFOBU_1_Tx_Mux/1(Vehicle_Type)
  Ground_2/1 -> RFOBU_1_Tx_Mux/6(spare_5)
  Ground_3/1 -> RFOBU_1_Tx_Mux/7(spare_6)
  Ground_4/1 -> RFOBU_1_Tx_Mux/8(spare_7)
  Ground_5/1 -> RFOBU_1_Tx_Mux/9(spare_8)
  Ground_6/1 -> RFOBU_1_Tx_Mux/10(spare_9)
  Ground_7/1 -> RFOBU_1_Tx_Mux/11(spare_10)
  Ground_8/1 -> RFOBU_1_Tx_Mux/12(spare_11)
  Ground_9/1 -> RFOBU_1_Tx_Mux/13(spare_12)
  Ground_10/1 -> RFOBU_1_Tx_Mux/14(spare_13)
  Ground_11/1 -> RFOBU_1_Tx_Mux/15(spare_14)
  Ground_12/1 -> RFOBU_1_Tx_Mux/16(spare_15)
  SELF_Demux/1(x [m]) -> Terminator_17/1
  SELF_Demux/2(y [m]) -> Terminator_18/1
  SELF_Demux/3(z [m]) -> Terminator_19/1
  SELF_Demux/4(rotx [deg]) -> Terminator_20/1
  SELF_Demux/5(roty [deg]) -> Terminator_21/1
  SELF_Demux/6(rotz [deg]) -> Terminator_22/1
  SELF_Demux/7(GPS lat [deg]) -> Terminator_23/1
  SELF_Demux/8(GPS long [deg]) -> Terminator_24/1
  SELF_Demux/9(GPS alt [m]) -> Terminator_25/1
  SELF_Demux/10(velocity [m/s]) -> Terminator_26/1
  SELF_Demux/11(heading [deg]) -> Terminator_27/1
  SELF_Demux/12(yaw rate [deg/s]) -> Terminator_28/1

== system Demo_TollSystem_cs/RFBeacon_1_Rx ==
  Selector : Selector  IndexMode=Zero-based  IndexOptions=Starting index (dialog)  Indices=PortIndex  OutputSizes=PortWidth(1)
  U : Outport
  wires:
  [SimCoreSensors] -> Selector/1
  Selector/1 -> U/1

== system Demo_TollSystem_cs/RFBeacon_1_Tx ==
  Y : Inport  SampleTime=TimeStep
  Assignment : Assignment  IndexMode=Zero-based  SampleTime=TimeStep  IndexOptions=Starting index (dialog)  Indices=PortIndex  OutputSizes=[1 1]
  Data Store Read : DataStoreRead  DataStoreName=SimCoreActuators  SampleTime=TimeStep
  Data Store Write : DataStoreWrite  DataStoreName=SimCoreActuators
  wires:
  Y/1 -> Assignment/2
  Data Store Read/1 -> Assignment/1
  Assignment/1 -> Data Store Write/1

== system Demo_TollSystem_cs/RFBeacon_2_Rx ==
  Selector : Selector  IndexMode=Zero-based  IndexOptions=Starting index (dialog)  Indices=PortIndex  OutputSizes=PortWidth(1)
  U : Outport
  wires:
  [SimCoreSensors] -> Selector/1
  Selector/1 -> U/1

== system Demo_TollSystem_cs/RFBeacon_2_Tx ==
  Y : Inport  SampleTime=TimeStep
  Assignment : Assignment  IndexMode=Zero-based  SampleTime=TimeStep  IndexOptions=Starting index (dialog)  Indices=PortIndex  OutputSizes=[1 1]
  Data Store Read : DataStoreRead  DataStoreName=SimCoreActuators  SampleTime=TimeStep
  Data Store Write : DataStoreWrite  DataStoreName=SimCoreActuators
  wires:
  Y/1 -> Assignment/2
  Data Store Read/1 -> Assignment/1
  Assignment/1 -> Data Store Write/1

== system Demo_TollSystem_cs/RFBeacon_3_Rx ==
  Selector : Selector  IndexMode=Zero-based  IndexOptions=Starting index (dialog)  Indices=PortIndex  OutputSizes=PortWidth(1)
  U : Outport
  wires:
  [SimCoreSensors] -> Selector/1
  Selector/1 -> U/1

== system Demo_TollSystem_cs/RFBeacon_3_Tx ==
  Y : Inport  SampleTime=TimeStep
  Assignment : Assignment  IndexMode=Zero-based  SampleTime=TimeStep  IndexOptions=Starting index (dialog)  Indices=PortIndex  OutputSizes=[1 1]
  Data Store Read : DataStoreRead  DataStoreName=SimCoreActuators  SampleTime=TimeStep
  Data Store Write : DataStoreWrite  DataStoreName=SimCoreActuators
  wires:
  Y/1 -> Assignment/2
  Data Store Read/1 -> Assignment/1
  Assignment/1 -> Data Store Write/1

== system Demo_TollSystem_cs/RFOBU_1_Rx ==
  Selector : Selector  IndexMode=Zero-based  IndexOptions=Starting index (dialog)  Indices=PortIndex  OutputSizes=PortWidth(1)
  U : Outport
  wires:
  Selector/1 -> U/1
  [SimCoreSensors] -> Selector/1

== system Demo_TollSystem_cs/RFOBU_1_Tx ==
  Y : Inport  SampleTime=TimeStep
  Assignment : Assignment  IndexMode=Zero-based  SampleTime=TimeStep  IndexOptions=Starting index (dialog)  Indices=PortIndex  OutputSizes=[1 1]
  Data Store Read : DataStoreRead  DataStoreName=SimCoreActuators  SampleTime=TimeStep
  Data Store Write : DataStoreWrite  DataStoreName=SimCoreActuators
  wires:
  Assignment/1 -> Data Store Write/1
  Data Store Read/1 -> Assignment/1
  Y/1 -> Assignment/2

== system Demo_TollSystem_cs/SELF_Mazda_RX8_1 ==
  Selector : Selector  IndexMode=Zero-based  IndexOptions=Starting index (dialog)  Indices=PortIndex  OutputSizes=PortWidth(1)
  U : Outport
  wires:
  Selector/1 -> U/1
  [SimCoreSensors] -> Selector/1

== system Demo_TollSystem_cs/STATE_Mazda_RX8_1 ==
  State : Inport  SampleTime=TimeStep
  Acceleration : Subsystem  mask(ToSensorWorld){PortName=Acceleration_Mazda_RX8_1, PortIndex=6, PortWidth=3, TimeStep=1/20}
      mask prompts: PortName "Port Name [-]"; PortIndex "Index [-]"; PortWidth "Port Dimensions [-]"; TimeStep "Upload Period [s]"
      mask help: Sends signal(s) from Simulink to the Sensor World
      mask Help:
      | Sends signal(s) from Simulink to the Sensor World.
      | 
      | - Port Name [-]: specifies the name of the output terminal of the Simulink block.
      | - Index [-]: specifies the start position in the output vector sent to the Sensor World
      | - Port dimensions [-]: specifies the width (number of scalars) of the output port
      | - Upload period [s]: specifies the upload period (in seconds) of the port.
      mask Display: port_label('input', 1, PortName)
  Demux : Demux  Outputs=5
  Position : Subsystem  mask(ToSensorWorld){PortName=Position_Mazda_RX8_1, PortIndex=0, PortWidth=3, TimeStep=1/20}
      mask prompts: PortName "Port Name [-]"; PortIndex "Index [-]"; PortWidth "Port Dimensions [-]"; TimeStep "Upload Period [s]"
      mask help: Sends signal(s) from Simulink to the Sensor World
      mask Help:
      | Sends signal(s) from Simulink to the Sensor World.
      | 
      | - Port Name [-]: specifies the name of the output terminal of the Simulink block.
      | - Index [-]: specifies the start position in the output vector sent to the Sensor World
      | - Port dimensions [-]: specifies the width (number of scalars) of the output port
      | - Upload period [s]: specifies the upload period (in seconds) of the port.
      mask Display: port_label('input', 1, PortName)
  RPY : Subsystem  mask(ToSensorWorld){PortName=RPY_Mazda_RX8_1, PortIndex=9, PortWidth=3, TimeStep=1/20}
      mask prompts: PortName "Port Name [-]"; PortIndex "Index [-]"; PortWidth "Port Dimensions [-]"; TimeStep "Upload Period [s]"
      mask help: Sends signal(s) from Simulink to the Sensor World
      mask Help:
      | Sends signal(s) from Simulink to the Sensor World.
      | 
      | - Port Name [-]: specifies the name of the output terminal of the Simulink block.
      | - Index [-]: specifies the start position in the output vector sent to the Sensor World
      | - Port dimensions [-]: specifies the width (number of scalars) of the output port
      | - Upload period [s]: specifies the upload period (in seconds) of the port.
      mask Display: port_label('input', 1, PortName)
  Velocity : Subsystem  mask(ToSensorWorld){PortName=Velocity_Mazda_RX8_1, PortIndex=3, PortWidth=3, TimeStep=1/20}
      mask prompts: PortName "Port Name [-]"; PortIndex "Index [-]"; PortWidth "Port Dimensions [-]"; TimeStep "Upload Period [s]"
      mask help: Sends signal(s) from Simulink to the Sensor World
      mask Help:
      | Sends signal(s) from Simulink to the Sensor World.
      | 
      | - Port Name [-]: specifies the name of the output terminal of the Simulink block.
      | - Index [-]: specifies the start position in the output vector sent to the Sensor World
      | - Port dimensions [-]: specifies the width (number of scalars) of the output port
      | - Upload period [s]: specifies the upload period (in seconds) of the port.
      mask Display: port_label('input', 1, PortName)
  iniBODYAngles wrtVEH [rad] : Constant  Value=[Roll0 Pitch0 0]  SampleTime=TimeStep
  iniVEHAngles wrtGLOB [rad] : Constant  Value=[0 0 Yaw0]  SampleTime=TimeStep
  iniVEHposition wrtGLOB [m] : Constant  Value=[x0 y0 z0]  SampleTime=TimeStep
  state2FullState : PreScanSimulinkLibrary/state2FullState  SystemSampleTime=-1
  velRPY : Subsystem  mask(ToSensorWorld){PortName=velRPY_Mazda_RX8_1, PortIndex=12, PortWidth=3, TimeStep=1/20}
      mask prompts: PortName "Port Name [-]"; PortIndex "Index [-]"; PortWidth "Port Dimensions [-]"; TimeStep "Upload Period [s]"
      mask help: Sends signal(s) from Simulink to the Sensor World
      mask Help:
      | Sends signal(s) from Simulink to the Sensor World.
      | 
      | - Port Name [-]: specifies the name of the output terminal of the Simulink block.
      | - Index [-]: specifies the start position in the output vector sent to the Sensor World
      | - Port dimensions [-]: specifies the width (number of scalars) of the output port
      | - Upload period [s]: specifies the upload period (in seconds) of the port.
      mask Display: port_label('input', 1, PortName)
  wires:
  Demux/5 -> velRPY/1(Y)
  Demux/4 -> RPY/1(Y)
  Demux/3 -> Acceleration/1(Y)
  Demux/2 -> Velocity/1(Y)
  Demux/1 -> Position/1(Y)
  State/1 -> state2FullState/1
  state2FullState/1 -> Demux/1
  iniVEHposition wrtGLOB [m]/1 -> state2FullState/2
  iniBODYAngles wrtVEH [rad]/1 -> state2FullState/3
  iniVEHAngles wrtGLOB [rad]/1 -> state2FullState/4

== system Demo_TollSystem_cs/SetActuators ==
  Bus Creator : BusCreator  Inputs=1
  Data Store Read : DataStoreRead  DataStoreName=SimCoreActuators  SampleTime=TimeStep
  SendActuators : M-S-Function  FunctionName=SendActuatorsBlock  Parameters=TimeStep NrOfActuators
  dummy : Outport
  tag scope: SimCoreInfo=global
  wires:
  Bus Creator/1 -> [SimCoreInfo]  "SimCore"
  SendActuators/2 -> Bus Creator/1  "ComputationTime[s]"
  SendActuators/1 -> dummy/1
  Data Store Read/1 -> SendActuators/1

== system Demo_TollSystem_cs/SimCoreInfo ==
  Bus Selector : BusSelector  OutputSignals=ComputationTime[s]
  Time : Scope
      settings: TimeRange=10  YMin=0  YMax=0.5  SaveName=ComputationTime
  wires:
  Bus Selector/1 -> Time/1  "<ComputationTime[s]>"
  [SimCoreInfo] -> Bus Selector/1

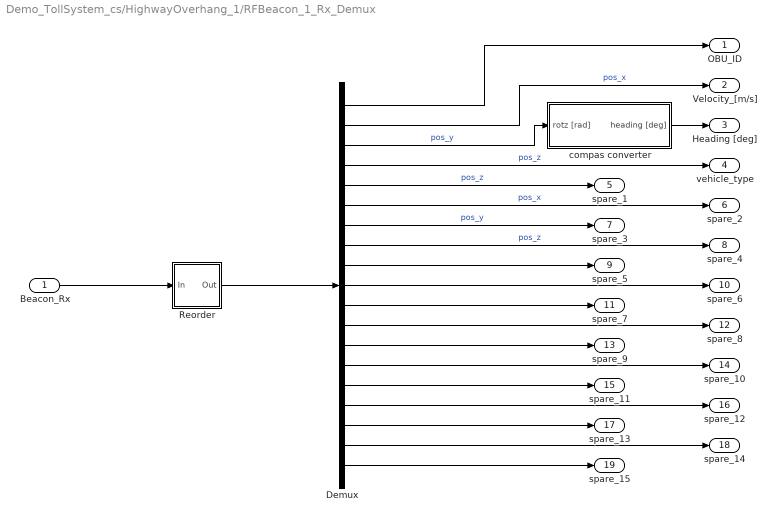
== system Demo_TollSystem_cs/HighwayOverhang_1/RFBeacon_1_Rx_Demux ==
  Beacon_Rx : Inport
  Demux : Demux  Outputs=19
  Reorder : Subsystem  mask(Output reorder block){NrOfOutputs=19, NrOfObjects=5}
      mask prompts: NrOfOutputs "Number Of Outputs [-]"; NrOfObjects "Number Of Objects [-]"
      mask help: Change output order from object based to output type based
      mask init:
      | InputPortWidth=NrOfObjects*NrOfOutputs;
      | Input=1:InputPortWidth;
      | ReshapedInput=reshape(Input,NrOfOutputs,NrOfObjects);
      | TransposedReshapedInput=transpose(ReshapedInput);
      | Elements=reshape(TransposedReshapedInput,length(Input),1);
  compas converter : Subsystem
  OBU_ID : Outport
  Velocity_[m/s] : Outport  Port=2
  Heading [deg] : Outport  Port=3
  vehicle_type : Outport  Port=4
  spare_1 : Outport  Port=5
  spare_2 : Outport  Port=6
  spare_3 : Outport  Port=7
  spare_4 : Outport  Port=8
  spare_5 : Outport  Port=9
  spare_6 : Outport  Port=10
  spare_7 : Outport  Port=11
  spare_8 : Outport  Port=12
  spare_9 : Outport  Port=13
  spare_10 : Outport  Port=14
  spare_11 : Outport  Port=15
  spare_12 : Outport  Port=16
  spare_13 : Outport  Port=17
  spare_14 : Outport  Port=18
  spare_15 : Outport  Port=19
  wires:
  compas converter/1(heading [deg]) -> Heading [deg]/1
  Demux/1 -> OBU_ID/1
  Demux/3 -> compas converter/1(rotz [rad])  "pos_y"
  Demux/2 -> Velocity_[m/s]/1  "pos_x"
  Reorder/1(Out) -> Demux/1
  Demux/5 -> spare_1/1  "pos_z"
  Demux/6 -> spare_2/1  "pos_x"
  Demux/7 -> spare_3/1  "pos_y"
  Demux/8 -> spare_4/1  "pos_z"
  Demux/9 -> spare_5/1
  Demux/10 -> spare_6/1
  Demux/11 -> spare_7/1
  Demux/12 -> spare_8/1
  Demux/13 -> spare_9/1
  Demux/14 -> spare_10/1
  Beacon_Rx/1 -> Reorder/1(In)
  Demux/4 -> vehicle_type/1  "pos_z"
  Demux/15 -> spare_11/1
  Demux/16 -> spare_12/1
  Demux/17 -> spare_13/1
  Demux/18 -> spare_14/1
  Demux/19 -> spare_15/1
